simulink model "EduardoApenasLMI"  (Simulink 8.2)
settings: Solver=ode4  SolverMode=SingleTasking  StartTime=0.0  StopTime=25  FixedStep=0.01  RelTol=1e-3
InitFcn:
  | Main;
values from neighbouring files (symbols this model uses):
  T = 0.5    [Main.m]
  xk0 = [-10; 0]    [x0.m]
undefined symbols (not defined in the file or in its folder): A, B, C, Cstate, Dstate
settings Model: Creator=Kawakami  LastModifiedBy=Eduardo
settings DataIOCC: LimitDataPoints=off  SaveOutput=off  SaveTime=off  TimeSaveName=t  SignalLoggingName=sigsOut
settings OptimizationCC: BooleanDataType=off
settings DebuggingCC: SaveWithParameterizedLinksMsg=none  SignalResolutionControl=TryResolveAllWithWarning  SolverPrmCheckMsg=none  MultiTaskDSMMsg=warning  MultiTaskCondExecSysMsg=none
settings HardwareCC: TargetUnknown=on
settings RTWCC: IncludeERTFirstTime=on

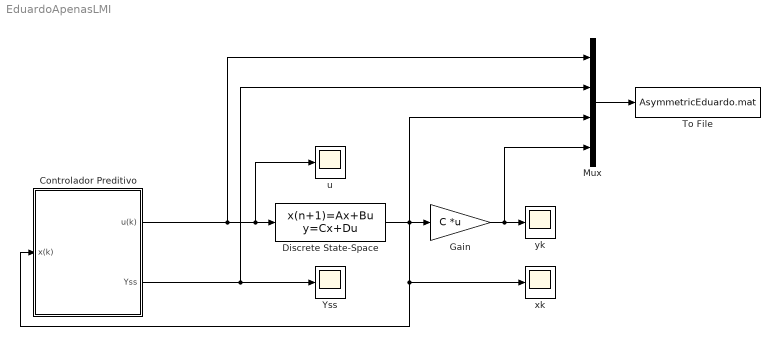
== system EduardoApenasLMI ==
  "Controlador Preditivo  " : Subsystem
  Discrete State-Space : DiscreteStateSpace  A=A{1}  B=B{1}  C=Cstate  D=Dstate  X0=xk0  SampleTime=T
  Gain : Gain  Gain=C  Multiplication=Matrix(K*u)
  Mux : Mux
  To File : ToFile  Filename=AsymmetricEduardo.mat  MatrixName=Eduardo  SampleTime=T
  Yss : Scope
      settings: TimeRange=10  YMin=-3e-06  YMax=1.1e-05  SaveName=ScopeData3
  u : Scope
      settings: TimeRange=10  YMin=-3e-06  YMax=1.1e-05
  xk : Scope
      settings: YMin=-1.25  YMax=2.25  SaveName=ScopeData2
  yk : Scope
      settings: YMin=-1.25  YMax=2.25
  wires:
  "Controlador Preditivo  "/1(u(k)) -> u/1, Discrete State-Space/1, Mux/1
  Discrete State-Space/1 -> Mux/3, Gain/1, xk/1, "Controlador Preditivo  "/1(x(k))
  Gain/1 -> Mux/4, yk/1
  "Controlador Preditivo  "/2(Yss) -> Yss/1, Mux/2
  Mux/1 -> To File/1

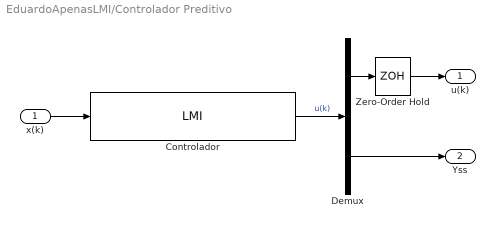
== system EduardoApenasLMI/Controlador Preditivo   ==
  x(k) : Inport
  Controlador : S-Function  FunctionName=LMI  Parameters=A, B, C, H, S, Smeio, R, Rmeio, Umax, Y, at, rho, T  EnableBusSupport=off
  Demux : Demux  Outputs=2
  Zero-Order Hold : ZeroOrderHold  SampleTime=T
  u(k) : Outport
  Yss : Outport  Port=2
  wires:
  Zero-Order Hold/1 -> u(k)/1
  x(k)/1 -> Controlador/1
  Controlador/1 -> Demux/1  "u(k)"
  Demux/1 -> Zero-Order Hold/1
  Demux/2 -> Yss/1
